simulink model "Project6"  (R2018b)
settings: Solver=ode4  StartTime=0.0  StopTime=1e-4  FixedStep=10e-12  RelTol=1e-3
libraries: simulink x2
settings Model: Creator=Samjat Chan  LastModifiedBy=Samjat Chan

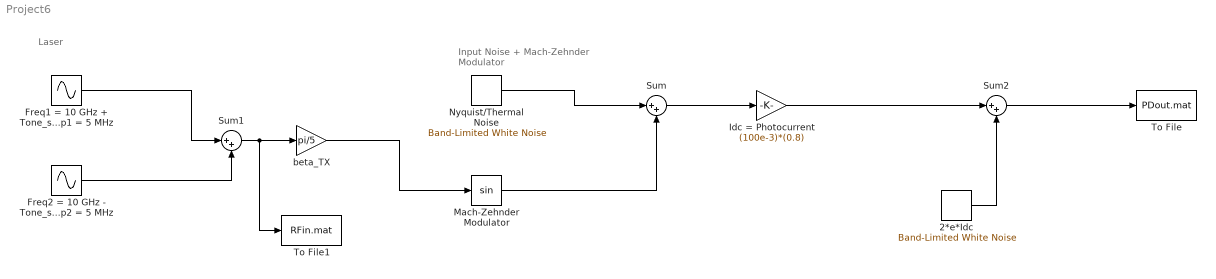
== system Project6 ==
  note: Input Noise + Mach-Zehnder Modulator
  note: Laser
  2*e*Idc : simulink/Sources/Band-Limited White Noise  Cov=2*(1.6e-19)*0.08  Ts=10e-12  seed=[23341]
  Freq1 = 10 GHz + Tone_sep1 Amp1 = 1 V Tone_sep1 = 5 MHz : Sin  Frequency=(10e9+10e6)*2*pi  SampleTime=10e-12
  Freq2 = 10 GHz - Tone_sep2 Amp2 = 1 V Tone_sep2 = 5 MHz : Sin  Frequency=(10e9-10e6)*2*pi  SampleTime=10e-12
  Idc = Photocurrent : Gain  Gain=(100e-3)*(0.8)
  Mach-Zehnder Modulator : Trigonometry
  Nyquist/Thermal Noise : simulink/Sources/Band-Limited White Noise  Cov=[(1.38e-23)*(300)*50]  Ts=10e-12  seed=[23341]
  Sum : Sum  Inputs=|++
  Sum1 : Sum  Inputs=|++
  Sum2 : Sum  Inputs=|++
  To File : ToFile  Filename=PDout.mat  MatrixName=pdout
  To File1 : ToFile  Filename=RFin.mat  MatrixName=rfin
  beta_TX : Gain  Gain=pi/5
  wires:
  Sum/1 -> Idc = Photocurrent/1
  Sum1/1 -> To File1/1, beta_TX/1
  Freq1 = 10 GHz + Tone_sep1 Amp1 = 1 V Tone_sep1 = 5 MHz/1 -> Sum1/1
  Freq2 = 10 GHz - Tone_sep2 Amp2 = 1 V Tone_sep2 = 5 MHz/1 -> Sum1/2
  Nyquist/Thermal Noise/1 -> Sum/1
  beta_TX/1 -> Mach-Zehnder Modulator/1
  2*e*Idc/1 -> Sum2/2
  Sum2/1 -> To File/1
  Idc = Photocurrent/1 -> Sum2/1
  Mach-Zehnder Modulator/1 -> Sum/2
